simulink model "Robot_KinematicsSim_2019b1"  (R2020b)
settings: Solver=VariableStepAuto  StartTime=0.0  StopTime=1000  RelTol=1e-3  EnableMultiTasking=on
model workspace (MAT data in the model file):
  Ts = 0.01
  Xmax = 500
  Ymax = 500
values from neighbouring files (symbols this model uses):
  animation_update_interval = C*h_fixed    [setup.m]
  enable_CG_trace = 1    [setup.m]
  enable_rearAxle_trace = 0    [setup.m]
  plotAxisLimitMode = 0    [setup.m]
  plotAxisLimits = plotAxisLimits    [graphical_development.m]    (also in setup.m = [-3 5 -3 6]*3)
  save_anim_frames = 0    [setup.m]
  vehicle_length = 5    [setup.m]
  vehicle_width = 2    [setup.m]
undefined symbols (not defined in the file or in its folder): datetime, DiscIntNeverNeededParam
libraries: arduinolib x21, simulink x4, pid_lib x2
(part 1 of 2)
settings Model: SimulationMode=accelerator  SILPILModeSetting=veronly  PacingRate=89  ExtModeTrigDuration=2  Creator=pc world  LastModifiedBy=Omen
settings SolverCC: AutoInsertRateTranBlk=on
settings OptimizationCC: EnhancedBackFolding=on  PassReuseOutputArgsAs=Individual arguments  ZeroExternalMemoryAtStartup=off  ZeroInternalMemoryAtStartup=off  MaxStackSize=64  OptimizeBlockOrder=speed  DifferentSizesBufferReuse=on  OptimizationCustomize=off  EfficientTunableParamExpr=on
settings DebuggingCC: ParameterTunabilityLossMsg=error  SFUnexpectedBacktrackingDiag=warning  SFNoUnconditionalDefaultTransitionDiag=warning  UnderSpecifiedDimensionMsg=warning
settings HardwareCC: ProdBitPerInt=16  ProdBitPerPointer=16  ProdBitPerSizeT=16  ProdBitPerPtrDiffT=16  ProdLargestAtomicFloat=None  ProdWordSize=8  ProdHWDeviceType=Atmel->AVR
settings SFSimCC: MATLABDynamicMemAlloc=off
settings RTWCC: Description=Embedded Coder  SystemTargetFile=ert.tlc  HardwareBoard=Arduino Uno  TemplateMakefile=ert_default_tmf  GenerateReport=on  Toolchain=Arduino AVR  BuildConfiguration=Faster Runs  LaunchReport=on
settings CodeAppCC: ForceParamTrailComments=on  IgnoreCustomStorageClasses=off  OperatorAnnotations=on  SimulinkDataObjDesc=on  SFDataObjDesc=on  InsertBlockDesc=on
settings ERTTargetCC: SupportContinuousTime=on  SupportVariableSizeSignals=on  ExtMode=on  ExtModeStaticAllocSize=250  ExtModeMexArgs='127.0.0.1' 0 17725

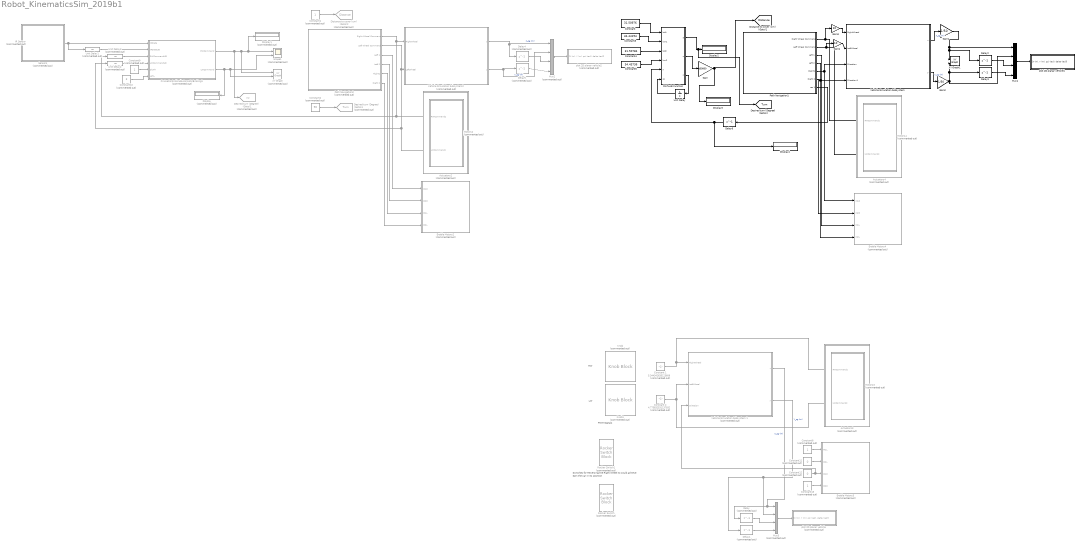
== system Robot_KinematicsSim_2019b1 ==
  note: PWM Signals
  note: RW
  note: LW
  note: Switches for Reversing the Right Wheel
      | to could achieve Spin the car in its position
  Actuators2 : Subsystem  Commented=on
  Actuators3 : Subsystem  Commented=on
  Actuators4 : Subsystem  Commented=on
  Constant : Constant  Value=31.50976
  Constant 1 : Constant  Commented=on  Value=5.344342635123609
  Constant 2 : Constant  Commented=on  Value=4.775832531137932
  Constant1 : Constant  Commented=on
  Constant10 : Constant  Commented=on  Value=3  OutDataTypeStr=double  SampleTime=Ts
  Constant11 : Constant  Commented=on  Value=0
  Constant12 : Constant  Commented=on  Value=0
  Constant13 : Constant  Commented=on
  Constant2 : Constant  Commented=on  Value=90
  Constant3 : Constant  Value=34.44194
  Constant4 : Constant  Value=31.50784
  Constant5 : Constant  Value=34.43736
  Constant8 : Constant  Commented=on
  Constant9 : Constant  Commented=on  OutDataTypeStr=double  SampleTime=Ts
  CruiseControlAndAutomaticBraking1 : Stateflow chart  Commented=on  TreatAsAtomicUnit=on
  Delay{,1,4..5} (4 alike) : Delay  Commented=on  DelayLength=1
  Delay2 : Delay  DelayLength=1
  Delay3 : Delay  DelayLength=1
  Delay6 : Delay  DelayLength=1
  Desired turn (Degree) (Goto)1 : Goto  Commented=on  GotoTag=rw  TagVisibility=global
  Desired turn (Degree) (Goto)3 : Goto  Commented=on  GotoTag=Turn  TagVisibility=global
  Display : Display  Commented=on
  Display1 : Display  Commented=on
  Display2 : Display
  Display3 : Display
  Display4 : Display
  Distance to cover (cm) (Goto)2 : Goto  Commented=on  GotoTag=Distance  TagVisibility=global
  Enable Motors2 : Subsystem  Commented=on
  Enable Motors3 : Subsystem  Commented=on
  Enable Motors4 : Subsystem  Commented=on
  Gain : Gain  Gain=100000
  Gain1 : Gain  Gain=1/50
  Gain2 : Gain  Gain=1/50
  Gain3 : Gain  Gain=10
  Gain4 : Gain  Gain=10
  IR Sensor : Subsystem  Commented=on
  Knob : KnobBlock  Commented=on  ScaleMax=10
  Knob1 : KnobBlock  Commented=on  ScaleMax=10
  MATLAB Function : MATLAB Function  TreatAsAtomicUnit=on
  Motors2 : Subsystem  Commented=on
  Motors3 : Subsystem  Commented=on
  Motors4 : Subsystem  Commented=on
  Mux1 : Mux
  Mux2 : Mux  Commented=on
  Mux3 : Mux  Commented=on
  Path Navigation1 : Subsystem
  Path Navigation2 : Subsystem  Commented=on
  Rocker Switch : RockerSwitchBlock  Commented=on
      settings: Values={{'Off', 'On'}, [0 1]}
  Rocker Switch1 : RockerSwitchBlock  Commented=on
      settings: Values={{'Off', 'On'}, [0 1]}
  Scope1 : Scope  Commented=on  NumInputPorts=2
  Sensors : Subsystem  Commented=on
  Unit Delay : UnitDelay  SampleTime=-1  HasFrameUpgradeWarning=on
  Unit Delay1 : UnitDelay  Commented=on  SampleTime=0.5  HasFrameUpgradeWarning=on
  Unit Delay2 : UnitDelay  Commented=on  SampleTime=0.5  HasFrameUpgradeWarning=on
  Unit Delay3 : UnitDelay  Commented=on  SampleTime=0.5  HasFrameUpgradeWarning=on
  "Vehicle Simulation Subsystem " : Subsystem
  Vehicle Simulation Subsystem 1 : Subsystem  Commented=on
  Vehicle Simulation Subsystem2 : Subsystem  Commented=on
  XY Graph : simulink/Sinks/XY Graph  Commented=on  xmin=-500  xmax=500  ymin=-500  ymax=500  st=0.05
  XY Graph1 : simulink/Sinks/XY Graph  xmin=-1000  xmax=1000  ymin=-1000  ymax=1000  st=0.05
  plot 2D planar vehicle : Subsystem  Commented=on  mask(6DoF Animation){axisMode=plotAxisLimitMode, ax=plotAxisLimits, Ts=animation_update_interval, enable_CG_trace=enable_CG_trace, enable_rearAxle_trace=enable_rearAxle_trace, save_anim_frames=save_anim_frames, anim_frame_name_str=char(datetime('now','Format','yyyy-MM-dd_HH_mm_ss')), L=vehicle_length, W=vehicle_width}
      mask prompts: axisMode "Axis Mode (0->auto, 1->fixed, BOTH use Axes Limits below)"; ax "Axes limits [xmin xmax ymin ymax] (m):"; Ts "Time interval between updates (s):"; enable_CG_trace "Enable vehicle CG trace? (0/1)"; enable_rearAxle_trace "Enable rear axle trace? (0/1)"; save_anim_frames "Save animaton frames? (0/1)"; anim_frame_name_str "Animation sequence name (if save frames==1)"; L "Vehicle length (m)"; W "Vehicle width (m)"
      mask help:
      | Create a 2D animated view of a steering vehicle model with tires.
      |
      | Marc Compere
      | CompereM@saic.com
      | created : 22 August 2002
      | modified: 28 Dec 2015
      mask init:
      | Config.axisMode=axisMode;
      | Config.ax=ax;
      | Config.Ts=Ts;
      | Config.enable_CG_trace=enable_CG_trace;
      | Config.enable_rearAxle_trace=enable_rearAxle_trace;
      | Config.save_anim_frames=save_anim_frames;
      | Config.anim_frame_name_str=anim_frame_name_str;
      | Config.L=L;
      | Config.W=W;
      mask Help:
      | <p>This block generates a 3 dimensional display of a simulation trajectory, with the craft orientation displayed during flight</p>
      | 
      | <p>There are two inputs to this block, Position and Euler.  These inputs contain more than one signal as described below.</p>
      | 
      | <p><H4>Block Vector Input - Position</H4>
      | <ul>
      | <li>X Position</li>
      | <li>Y Position</li>
      | <li>Z Position</li>
      | </ul>
      | </p>
      | 
      | <p><H4>Block Vector Input - Euler</H4>
      |     <ul>
      |     <li>Roll Attitude</li>
      |     <li>Pitch Attitude</li>
      |     <li>Yaw Attitude</li>
      |    </ul>
      |    </p>
  plot 2D planar vehicle1 : Subsystem  mask(6DoF Animation){axisMode=plotAxisLimitMode, ax=[-500 500 -500 500], Ts=animation_update_interval, enable_CG_trace=enable_CG_trace, enable_rearAxle_trace=enable_rearAxle_trace, save_anim_frames=save_anim_frames, anim_frame_name_str=char(datetime('now','Format','yyyy-MM-dd_HH_mm_ss')), L=vehicle_length, W=vehicle_width}
      mask prompts: axisMode "Axis Mode (0->auto, 1->fixed, BOTH use Axes Limits below)"; ax "Axes limits [xmin xmax ymin ymax] (m):"; Ts "Time interval between updates (s):"; enable_CG_trace "Enable vehicle CG trace? (0/1)"; enable_rearAxle_trace "Enable rear axle trace? (0/1)"; save_anim_frames "Save animaton frames? (0/1)"; anim_frame_name_str "Animation sequence name (if save frames==1)"; L "Vehicle length (m)"; W "Vehicle width (m)"
      mask help:
      | Create a 2D animated view of a steering vehicle model with tires.
      |
      | Marc Compere
      | CompereM@saic.com
      | created : 22 August 2002
      | modified: 28 Dec 2015
      mask init: same as Robot_KinematicsSim_2019b1/plot 2D planar vehicle
      mask Help:
      | <p>This block generates a 3 dimensional display of a simulation trajectory, with the craft orientation displayed during flight</p>
      | 
      | <p>There are two inputs to this block, Position and Euler.  These inputs contain more than one signal as described below.</p>
      | 
      | <p><H4>Block Vector Input - Position</H4>
      | <ul>
      | <li>X Position</li>
      | <li>Y Position</li>
      | <li>Z Position</li>
      | </ul>
      | </p>
      | 
      | <p><H4>Block Vector Input - Euler</H4>
      |     <ul>
      |     <li>Roll Attitude</li>
      |     <li>Pitch Attitude</li>
      |     <li>Yaw Attitude</li>
      |    </ul>
      |    </p>
  plot 2D planar vehicle2 : Subsystem  Commented=on  mask(6DoF Animation){axisMode=plotAxisLimitMode, ax=plotAxisLimits, Ts=animation_update_interval, enable_CG_trace=enable_CG_trace, enable_rearAxle_trace=enable_rearAxle_trace, save_anim_frames=save_anim_frames, anim_frame_name_str=char(datetime('now','Format','yyyy-MM-dd_HH_mm_ss')), L=vehicle_length, W=vehicle_width}
      mask prompts: axisMode "Axis Mode (0->auto, 1->fixed, BOTH use Axes Limits below)"; ax "Axes limits [xmin xmax ymin ymax] (m):"; Ts "Time interval between updates (s):"; enable_CG_trace "Enable vehicle CG trace? (0/1)"; enable_rearAxle_trace "Enable rear axle trace? (0/1)"; save_anim_frames "Save animaton frames? (0/1)"; anim_frame_name_str "Animation sequence name (if save frames==1)"; L "Vehicle length (m)"; W "Vehicle width (m)"
      mask help:
      | Create a 2D animated view of a steering vehicle model with tires.
      |
      | Marc Compere
      | CompereM@saic.com
      | created : 22 August 2002
      | modified: 28 Dec 2015
      mask init: same as Robot_KinematicsSim_2019b1/plot 2D planar vehicle
      mask Help:
      | <p>This block generates a 3 dimensional display of a simulation trajectory, with the craft orientation displayed during flight</p>
      | 
      | <p>There are two inputs to this block, Position and Euler.  These inputs contain more than one signal as described below.</p>
      | 
      | <p><H4>Block Vector Input - Position</H4>
      | <ul>
      | <li>X Position</li>
      | <li>Y Position</li>
      | <li>Z Position</li>
      | </ul>
      | </p>
      | 
      | <p><H4>Block Vector Input - Euler</H4>
      |     <ul>
      |     <li>Roll Attitude</li>
      |     <li>Pitch Attitude</li>
      |     <li>Yaw Attitude</li>
      |    </ul>
      |    </p>
  tag scope: Distance=global, Turn=global
  wires:
  Constant 1/1 -> Motors3/1(RWCommands), Vehicle Simulation Subsystem 1/1(RightWheel)
  Constant 2/1 -> Motors3/2(LWCommands), Vehicle Simulation Subsystem 1/2(LeftWheel)
  CruiseControlAndAutomaticBraking1/2(LWCommand) -> Scope1/2, XY Graph/2, Display/1
  CruiseControlAndAutomaticBraking1/1(RWCommand) -> Desired turn (Degree) (Goto)1/1, Scope1/1, Display1/1, XY Graph/1
  Unit Delay1/1 -> CruiseControlAndAutomaticBraking1/2(IRDataUD)
  Constant10/1 -> CruiseControlAndAutomaticBraking1/6(IRTh)
  IR Sensor/1(IRSensorMeasurement) -> Unit Delay1/1, CruiseControlAndAutomaticBraking1/1(IRData)
  Constant9/1 -> CruiseControlAndAutomaticBraking1/5(DisTh)
  Unit Delay3/1 -> CruiseControlAndAutomaticBraking1/3(RWCommandUD)
  Unit Delay2/1 -> CruiseControlAndAutomaticBraking1/4(LWCommandUD)
  Constant12/1 -> Enable Motors3/3(IN1R), Vehicle Simulation Subsystem 1/3(Direction)
  Constant8/1 -> Enable Motors3/1(IN1L)
  Constant13/1 -> Enable Motors3/4(IN2R)
  Constant11/1 -> Enable Motors3/2(IN2L)
  Mux3/1 -> plot 2D planar vehicle/1("[X (m), Y (m), psi (rad), delta (rad)]")
  Delay1/1 -> Mux3/4
  Delay/1 -> Mux3/3
  Vehicle Simulation Subsystem 1/1(x) -> Mux3/1, Delay/1  "X_cg (m)"
  Vehicle Simulation Subsystem 1/2(y) -> Mux3/2, Delay1/1  "Y_cg (m)"
  MATLAB Function/1(a) -> [Turn], Display2/1
  Path Navigation1/2(Left Wheel Command) -> Gain4/1, Motors4/2(LWCommands)
  Path Navigation1/1(Right Wheel Command) -> Gain3/1, Motors4/1(RWCommands)
  Delay2/1 -> Mux1/3
  Mux1/1 -> plot 2D planar vehicle1/1("[X (m), Y (m), psi (rad), delta (rad)]")
  Mux2/1 -> plot 2D planar vehicle2/1("[X (m), Y (m), psi (rad), delta (rad)]")
  Delay5/1 -> Mux2/4
  Delay4/1 -> Mux2/3
  Vehicle Simulation Subsystem2/1(x) -> Mux2/1, Delay4/1  "X_cg (m)"
  Vehicle Simulation Subsystem2/2(y) -> Mux2/2, Delay5/1  "Y_cg (m)"
  Path Navigation2/1(Right Wheel Command) -> Vehicle Simulation Subsystem2/1(RightWheel), Motors2/1(RWCommands), Unit Delay3/1
  Path Navigation2/2(Left Wheel Command) -> Vehicle Simulation Subsystem2/2(LeftWheel), Unit Delay2/1, Motors2/2(LWCommands)
  Constant1/1 -> Distance to cover (cm) (Goto)2/1
  Constant2/1 -> Desired turn (Degree) (Goto)3/1
  Path Navigation2/3(Left 1) -> Enable Motors2/1(IN1R)
  Path Navigation2/4(Left 2) -> Enable Motors2/2(IN2R)
  Path Navigation2/5(Right1) -> Enable Motors2/3(IN1L)
  Path Navigation2/6(Right 2) -> Enable Motors2/4(IN2L)
  Delay3/1 -> Mux1/4
  Path Navigation1/5(Right1) -> Enable Motors4/1(IN1R), "Vehicle Simulation Subsystem "/3(Direction)
  Path Navigation1/3(Left 1) -> Enable Motors4/3(IN1L)
  Path Navigation1/4(Left 2) -> Enable Motors4/4(IN2L), "Vehicle Simulation Subsystem "/4(Direction1)
  Path Navigation1/6(Right 2) -> Enable Motors4/2(IN2R)
  Constant4/1 -> MATLAB Function/3(lat2)
  Constant5/1 -> MATLAB Function/4(lon2)
  Unit Delay/1 -> MATLAB Function/6(ss)
  MATLAB Function/3(s) -> Unit Delay/1
  Constant/1 -> MATLAB Function/1(lat1)
  Constant3/1 -> MATLAB Function/2(lon1)
  Path Navigation1/7(res 1) -> Delay6/1
  Delay6/1 -> Display4/1, MATLAB Function/5(n)
  MATLAB Function/2(c) -> Gain/1
  Gain/1 -> [Distance], Display3/1
  "Vehicle Simulation Subsystem "/1(x) -> Gain1/1  "X_cg (m)"
  Gain1/1 -> Mux1/1, XY Graph1/1, Delay2/1
  "Vehicle Simulation Subsystem "/2(y) -> Gain2/1  "Y_cg (m)"
  Gain2/1 -> Delay3/1, XY Graph1/2, Mux1/2
  Gain3/1 -> "Vehicle Simulation Subsystem "/1(RightWheel)
  Gain4/1 -> "Vehicle Simulation Subsystem "/2(LeftWheel)

== system Robot_KinematicsSim_2019b1/Actuators2 ==

== system Robot_KinematicsSim_2019b1/Actuators3 ==

== system Robot_KinematicsSim_2019b1/Actuators4 ==

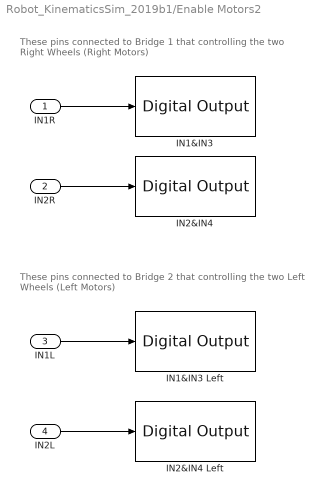
== system Robot_KinematicsSim_2019b1/Enable Motors2 ==
  note: These pins connected to Bridge 1 that
      | controlling the two Right Wheels (Right Motors)
  note: These pins connected to Bridge 2 that
      | controlling the two Left Wheels (Left Motors)
  IN1R : Inport
  IN2R : Inport  Port=2
  IN1L : Inport  Port=3
  IN2L : Inport  Port=4
  IN1&IN3 : arduinolib/Digital Output  pinNumber=12  Direction=output  blockPlatform=arduino
  IN1&IN3 Left : arduinolib/Digital Output  pinNumber=8  Direction=output  blockPlatform=arduino
  IN2&IN4 : arduinolib/Digital Output  pinNumber=4  Direction=output  blockPlatform=arduino
  IN2&IN4 Left : arduinolib/Digital Output  pinNumber=7  Direction=output  blockPlatform=arduino
  wires:
  IN2R/1 -> IN2&IN4/1
  IN1R/1 -> IN1&IN3/1
  IN1L/1 -> IN1&IN3 Left/1
  IN2L/1 -> IN2&IN4 Left/1

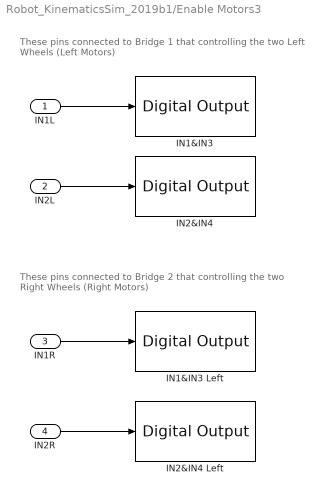
== system Robot_KinematicsSim_2019b1/Enable Motors3 ==
  note: These pins connected to Bridge 1 that
      | controlling the two Left Wheels (Left Motors)
  note: These pins connected to Bridge 2 that
      | controlling the two Right Wheels (Right Motors)
  IN1L : Inport
  IN2L : Inport  Port=2
  IN1R : Inport  Port=3
  IN2R : Inport  Port=4
  IN1&IN3 : arduinolib/Digital Output  pinNumber=12  Direction=output  blockPlatform=arduino
  IN1&IN3 Left : arduinolib/Digital Output  pinNumber=8  Direction=output  blockPlatform=arduino
  IN2&IN4 : arduinolib/Digital Output  pinNumber=4  Direction=output  blockPlatform=arduino
  IN2&IN4 Left : arduinolib/Digital Output  pinNumber=7  Direction=output  blockPlatform=arduino
  wires:
  IN2L/1 -> IN2&IN4/1
  IN1L/1 -> IN1&IN3/1
  IN1R/1 -> IN1&IN3 Left/1
  IN2R/1 -> IN2&IN4 Left/1

== system Robot_KinematicsSim_2019b1/Enable Motors4 ==
  note: These pins connected to Bridge 2 that
      | controlling the two Left Wheels (Left Motors)
  note: These pins connected to Bridge 1 that
      | controlling the two Right Wheels (Right Motors)
  IN1R : Inport
  IN2R : Inport  Port=2
  IN1L : Inport  Port=3
  IN2L : Inport  Port=4
  IN1&IN3 : arduinolib/Digital Output  pinNumber=12  Direction=output  blockPlatform=arduino
  IN1&IN3 Left : arduinolib/Digital Output  pinNumber=8  Direction=output  blockPlatform=arduino
  IN2&IN4 : arduinolib/Digital Output  pinNumber=4  Direction=output  blockPlatform=arduino
  IN2&IN4 Left : arduinolib/Digital Output  pinNumber=7  Direction=output  blockPlatform=arduino
  wires:
  IN2R/1 -> IN2&IN4 Left/1
  IN1R/1 -> IN1&IN3 Left/1
  IN1L/1 -> IN1&IN3/1
  IN2L/1 -> IN2&IN4/1

== system Robot_KinematicsSim_2019b1/IR Sensor ==
  "1-D Lookup Table " : Lookup_n-D  NumberOfTableDimensions=1  BreakpointsForDimension1=[440 470 500 550 700 850 1300 2250]  Table=[80 70 60 50 40 30 20 10]  ExtrapMethod=Clip  UseLastTableValue=on  InternalRulePriority=Speed  OutDataTypeStr=double  RndMeth=Simplest  InputSameDT=on
  "Analog Input " : arduinolib/Analog Input  pinNumber=4  ReadResultsOnly=off  ConversionTriggerSource=Software  ExternalTriggerType=uint32(0)  OutputDataType=uint16  EnableConversionCompleteNotify=off  EnableOuputStatus=off  SampleTime=Ts  blockPlatform=arduino
  Conversion to mV : Gain  Gain=3300/1023  OutDataTypeStr=int16
  "Discrete Transfer Fcn " : DiscreteTransferFcn  Numerator=0.5  Denominator=[1 -0.5]  OutDataTypeStr=int16
  Mux : Mux  Inputs=2
  Scope1 : Scope
  Scope2 : Scope
  IRSensorMeasurement : Outport
  wires:
  "Analog Input "/1 -> Conversion to mV/1
  Mux/1 -> Scope1/1
  Conversion to mV/1 -> "Discrete Transfer Fcn "/1, Mux/2  "raw Signal"
  "1-D Lookup Table "/1 -> Scope2/1, IRSensorMeasurement/1
  "Discrete Transfer Fcn "/1 -> Mux/1, "1-D Lookup Table "/1  "filtered Signal"

== system Robot_KinematicsSim_2019b1/Motors2 ==
  note: 10 is the maximum input from our model system
      | after scaling by 25.5 ,it will be equal 255
  RWCommands : Inport
  LWCommands : Inport  Port=2
  PWM to Enable the Left Bridge : arduinolib/PWM  pinNumber=6  frequencyType=Default  desiredFrequency=490.2  achievableFrequency=490.2
  PWM to Enable the Right Bridge : arduinolib/PWM  pinNumber=5  frequencyType=Default  desiredFrequency=490.2  achievableFrequency=490.2
  Scale1 : Gain  Gain=25.5
  Scale2 : Gain  Gain=25.5
  wires:
  LWCommands/1 -> Scale2/1
  RWCommands/1 -> Scale1/1
  Scale2/1 -> PWM to Enable the Left Bridge/1
  Scale1/1 -> PWM to Enable the Right Bridge/1

== system Robot_KinematicsSim_2019b1/Motors3 ==
  note: 10 is the maximum input from our model system
      | after scaling by 25.5 ,it will be equal 255
  RWCommands : Inport
  LWCommands : Inport  Port=2
  PWM to Enable the Left Bridge : arduinolib/PWM  pinNumber=6  frequencyType=Default  desiredFrequency=490.2  achievableFrequency=490.2
  PWM to Enable the Right Bridge : arduinolib/PWM  pinNumber=5  frequencyType=Default  desiredFrequency=490.2  achievableFrequency=490.2
  Scale1 : Gain  Gain=25.5
  Scale2 : Gain  Gain=25.5
  wires:
  LWCommands/1 -> Scale2/1
  RWCommands/1 -> Scale1/1
  Scale2/1 -> PWM to Enable the Left Bridge/1
  Scale1/1 -> PWM to Enable the Right Bridge/1

== system Robot_KinematicsSim_2019b1/Motors4 ==
  note: 10 is the maximum input from our model system
      | after scaling by 25.5 ,it will be equal 255
  RWCommands : Inport
  LWCommands : Inport  Port=2
  PWM to Enable the Left Bridge : arduinolib/PWM  pinNumber=6  frequencyType=Default  desiredFrequency=490.2  achievableFrequency=490.2
  PWM to Enable the Right Bridge : arduinolib/PWM  pinNumber=5  frequencyType=Default  desiredFrequency=490.2  achievableFrequency=490.2
  Scale1 : Gain  Gain=25.5
  Scale2 : Gain  Gain=25.5
  wires:
  Scale1/1 -> PWM to Enable the Right Bridge/1
  Scale2/1 -> PWM to Enable the Left Bridge/1
  RWCommands/1 -> Scale1/1
  LWCommands/1 -> Scale2/1

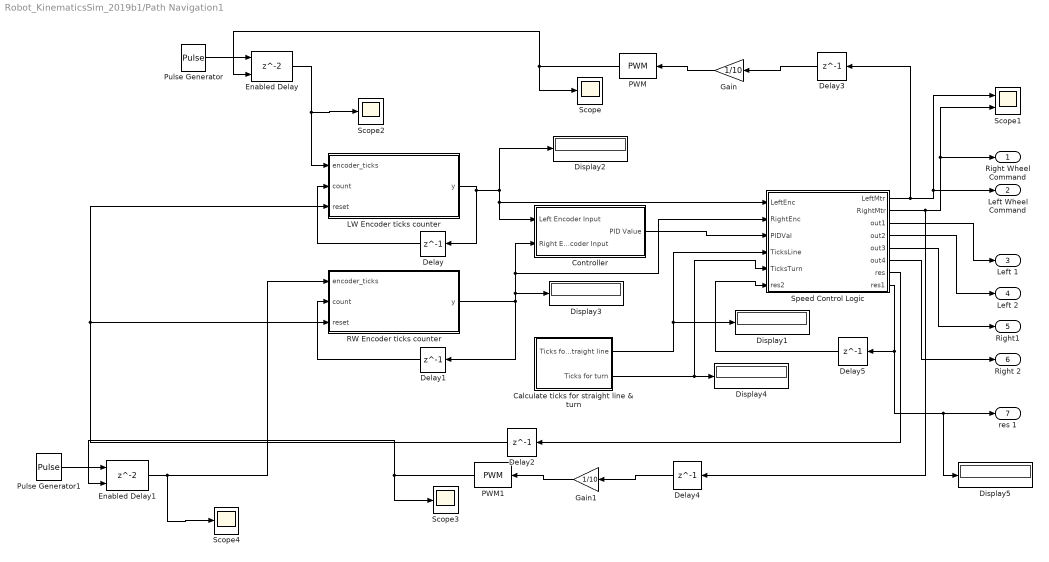
== system Robot_KinematicsSim_2019b1/Path Navigation1 ==
  Calculate ticks for straight line & turn : Subsystem
  Controller : Subsystem
  Delay{,1..2,5} (4 alike) : Delay  DelayLength=1  InitialCondition=0
  Delay3 : Delay  DelayLength=1
  Delay4 : Delay  DelayLength=1
  Display{1..5} (5 alike) : Display
  Enabled Delay : Delay  ShowEnablePort=on
      settings: InputPortMap=u0,e6
  Enabled Delay1 : Delay  ShowEnablePort=on
      settings: InputPortMap=u0,e6
  Gain : Gain  Gain=1/10
  Gain1 : Gain  Gain=1/10
  LW Encoder ticks counter : MATLAB Function  TreatAsAtomicUnit=on
  PWM : simulink/Discontinuities/PWM  DisableCoverage=on  Period=1/100  DisallowZeroDutyCycle=off  RunAtFixedTimeIntervals=on  SampleTime=0.01
  PWM1 : simulink/Discontinuities/PWM  DisableCoverage=on  Period=1/100  DisallowZeroDutyCycle=off  RunAtFixedTimeIntervals=on  SampleTime=0.01
  Pulse Generator : DiscretePulseGenerator  PulseType=Time based  Period=1/1000  PulseWidth=10  SampleTime=6
  Pulse Generator1 : DiscretePulseGenerator  PulseType=Time based  Period=1/1000  PulseWidth=10  SampleTime=6
  RW Encoder ticks counter : MATLAB Function  TreatAsAtomicUnit=on
  Scope{,2..4} (4 alike) : Scope
  Scope1 : Scope  NumInputPorts=2
  Speed Control Logic : MATLAB Function  TreatAsAtomicUnit=on
      settings: CopyFcn=set_param(gcb, 'LinkStatus', 'none') ;
  Right Wheel Command : Outport
  Left Wheel Command : Outport  Port=2
  Left 1 : Outport  Port=3
  Left 2 : Outport  Port=4
  Right1 : Outport  Port=5
  Right 2 : Outport  Port=6
  res 1 : Outport  Port=7
  wires:
  Delay5/1 -> Speed Control Logic/6(res2)
  Speed Control Logic/6(out4) -> Right 2/1
  Speed Control Logic/5(out3) -> Right1/1
  Speed Control Logic/4(out2) -> Left 2/1
  Speed Control Logic/3(out1) -> Left 1/1
  Delay2/1 -> LW Encoder ticks counter/3(reset), RW Encoder ticks counter/3(reset)
  Speed Control Logic/7(res) -> Delay2/1
  Enabled Delay1/1 -> RW Encoder ticks counter/1(encoder_ticks), Scope4/1
  RW Encoder ticks counter/1(y) -> Display3/1, Speed Control Logic/2(RightEnc), Controller/2(Right Encoder Input), Delay1/1
  Delay1/1 -> RW Encoder ticks counter/2(count)
  Delay/1 -> LW Encoder ticks counter/2(count)
  LW Encoder ticks counter/1(y) -> Speed Control Logic/1(LeftEnc), Controller/1(Left Encoder Input), Display2/1, Delay/1
  Speed Control Logic/2(RightMtr) -> Delay4/1, Scope1/2, Right Wheel Command/1
  Calculate ticks for straight line & turn/1("Ticks for straight line ") -> Speed Control Logic/4(TicksLine), Display1/1
  Controller/1(PID Value) -> Speed Control Logic/3(PIDVal)
  Speed Control Logic/1(LeftMtr) -> Delay3/1, Left Wheel Command/1, Scope1/1
  Calculate ticks for straight line & turn/2(Ticks for turn) -> Display4/1, Speed Control Logic/5(TicksTurn)
  Speed Control Logic/8(res1) -> Delay5/1, Display5/1, res 1/1
  Enabled Delay/1 -> Scope2/1, LW Encoder ticks counter/1(encoder_ticks)
  Pulse Generator/1 -> Enabled Delay/1
  Gain/1 -> PWM/1
  PWM/1 -> Scope/1, Enabled Delay/2
  Delay3/1 -> Gain/1
  Gain1/1 -> PWM1/1
  Delay4/1 -> Gain1/1
  Pulse Generator1/1 -> Enabled Delay1/1
  PWM1/1 -> Scope3/1, Enabled Delay1/2

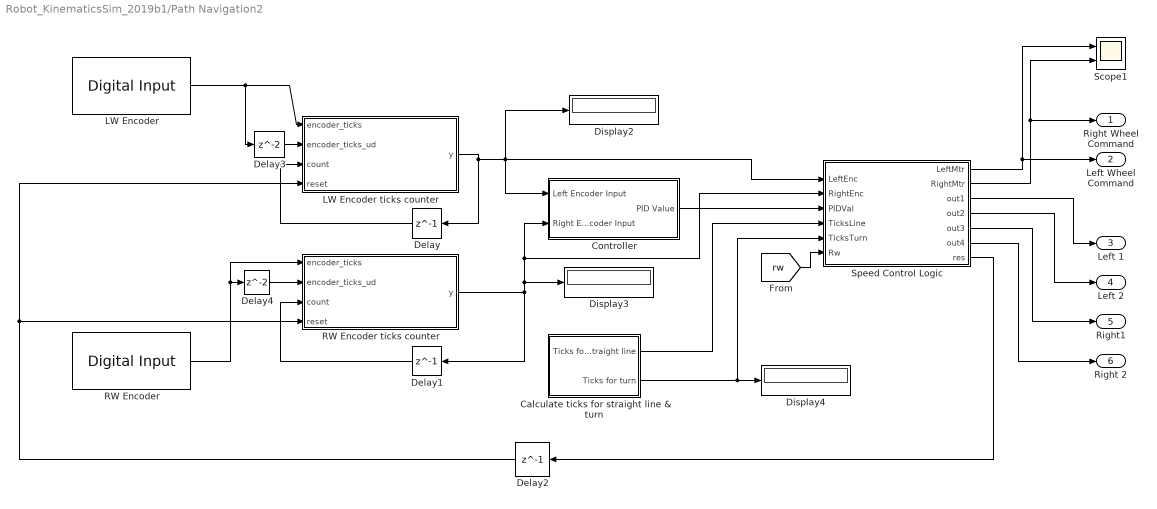
== system Robot_KinematicsSim_2019b1/Path Navigation2 ==
  Calculate ticks for straight line & turn : Subsystem
  Controller : Subsystem
  Delay : Delay  DelayLength=1  InitialCondition=0
  Delay1 : Delay  DelayLength=1  InitialCondition=0
  Delay2 : Delay  DelayLength=1  InitialCondition=0
  Delay3 : Delay  InitialCondition=0
  Delay4 : Delay  InitialCondition=0
  Display2 : Display
  Display3 : Display
  Display4 : Display
  LW Encoder : arduinolib/Digital Input  pinNumber=2  mode=Default  Direction=input  SampleTime=0.1  blockPlatform=arduino
  LW Encoder ticks counter : MATLAB Function  TreatAsAtomicUnit=on
  RW Encoder : arduinolib/Digital Input  pinNumber=3  mode=Default  Direction=input  SampleTime=0.1  blockPlatform=arduino
  RW Encoder ticks counter : MATLAB Function  TreatAsAtomicUnit=on
  Scope1 : Scope  NumInputPorts=2
  Speed Control Logic : MATLAB Function  TreatAsAtomicUnit=on
      settings: CopyFcn=set_param(gcb, 'LinkStatus', 'none') ;
  Right Wheel Command : Outport
  Left Wheel Command : Outport  Port=2
  Left 1 : Outport  Port=3
  Left 2 : Outport  Port=4
  Right1 : Outport  Port=5
  Right 2 : Outport  Port=6
  wires:
  Calculate ticks for straight line & turn/2(Ticks for turn) -> Speed Control Logic/5(TicksTurn), Display4/1
  Speed Control Logic/1(LeftMtr) -> Scope1/1, Left Wheel Command/1
  Controller/1(PID Value) -> Speed Control Logic/3(PIDVal)
  Calculate ticks for straight line & turn/1("Ticks for straight line ") -> Speed Control Logic/4(TicksLine)
  Speed Control Logic/2(RightMtr) -> Right Wheel Command/1, Scope1/2
  LW Encoder ticks counter/1(y) -> Delay/1, Controller/1(Left Encoder Input), Speed Control Logic/1(LeftEnc), Display2/1
  LW Encoder/1 -> Delay3/1, LW Encoder ticks counter/1(encoder_ticks)
  Delay/1 -> LW Encoder ticks counter/3(count)
  Delay1/1 -> RW Encoder ticks counter/3(count)
  RW Encoder ticks counter/1(y) -> Delay1/1, Controller/2(Right Encoder Input), Speed Control Logic/2(RightEnc), Display3/1
  RW Encoder/1 -> Delay4/1, RW Encoder ticks counter/1(encoder_ticks)
  Speed Control Logic/7(res) -> Delay2/1
  Delay2/1 -> RW Encoder ticks counter/4(reset), LW Encoder ticks counter/4(reset)
  Speed Control Logic/3(out1) -> Left 1/1
  Speed Control Logic/4(out2) -> Left 2/1
  Speed Control Logic/5(out3) -> Right1/1
  Speed Control Logic/6(out4) -> Right 2/1
  Delay3/1 -> LW Encoder ticks counter/2(encoder_ticks_ud)
  Delay4/1 -> RW Encoder ticks counter/2(encoder_ticks_ud)
  [rw] -> Speed Control Logic/6(Rw)

== system Robot_KinematicsSim_2019b1/Sensors ==

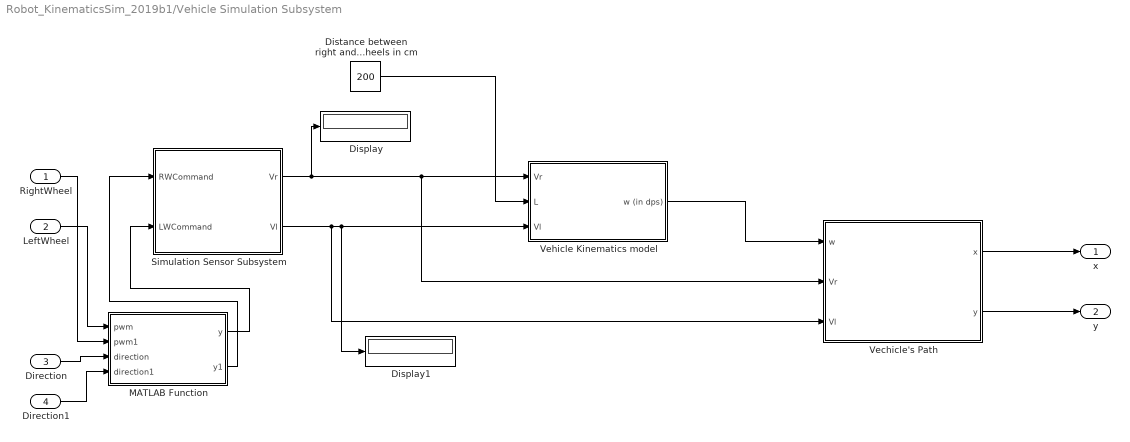
== system Robot_KinematicsSim_2019b1/Vehicle Simulation Subsystem  ==
  RightWheel : Inport
  LeftWheel : Inport  Port=2
  Direction : Inport  Port=3
  Direction1 : Inport  Port=4
  Display : Display
  Display1 : Display
  "Distance between right and left wheels in cm " : Constant  Value=200
  MATLAB Function : MATLAB Function  TreatAsAtomicUnit=on
  Simulation Sensor Subsystem : Subsystem
  "Vechicle's Path " : Subsystem
  "Vehicle Kinematics model " : Subsystem
  x : Outport
  y : Outport  Port=2
  wires:
  "Distance between right and left wheels in cm "/1 -> "Vehicle Kinematics model "/2(L)
  Simulation Sensor Subsystem/2(Vl) -> "Vehicle Kinematics model "/3("Vl "), Display1/1, "Vechicle's Path "/3(Vl)
  Simulation Sensor Subsystem/1(Vr) -> Display/1, "Vehicle Kinematics model "/1(Vr), "Vechicle's Path "/2(Vr)
  "Vechicle's Path "/2(y) -> y/1
  "Vechicle's Path "/1(x) -> x/1
  LeftWheel/1 -> MATLAB Function/1(pwm)
  MATLAB Function/1(y) -> Simulation Sensor Subsystem/2(LWCommand)
  Direction/1 -> MATLAB Function/3(direction)
  RightWheel/1 -> MATLAB Function/2(pwm1)
  MATLAB Function/2(y1) -> Simulation Sensor Subsystem/1(RWCommand)
  Direction1/1 -> MATLAB Function/4(direction1)
  "Vehicle Kinematics model "/1("w (in dps) ") -> "Vechicle's Path "/1(w)

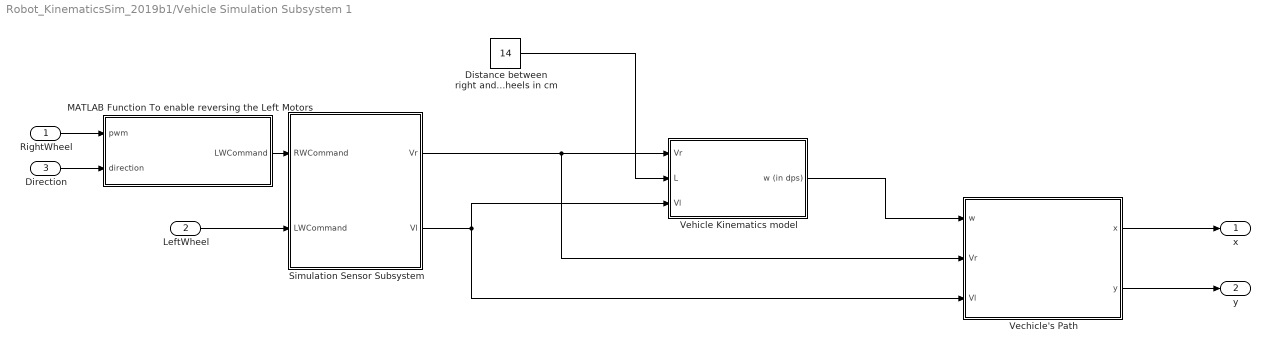
== system Robot_KinematicsSim_2019b1/Vehicle Simulation Subsystem 1 ==
  RightWheel : Inport
  LeftWheel : Inport  Port=2
  Direction : Inport  Port=3
  "Distance between right and left wheels in cm " : Constant  Value=14
  "MATLAB Function To enable reversing the Left Motors " : MATLAB Function  TreatAsAtomicUnit=on
  Simulation Sensor Subsystem : Subsystem
  "Vechicle's Path " : Subsystem
  "Vehicle Kinematics model " : Subsystem
  x : Outport
  y : Outport  Port=2
  wires:
  "Distance between right and left wheels in cm "/1 -> "Vehicle Kinematics model "/2(L)
  Simulation Sensor Subsystem/2(Vl) -> "Vechicle's Path "/3(Vl), "Vehicle Kinematics model "/3("Vl ")
  Simulation Sensor Subsystem/1(Vr) -> "Vechicle's Path "/2(Vr), "Vehicle Kinematics model "/1(Vr)
  "Vehicle Kinematics model "/1("w (in dps) ") -> "Vechicle's Path "/1(w)
  "Vechicle's Path "/2(y) -> y/1
  "Vechicle's Path "/1(x) -> x/1
  Direction/1 -> "MATLAB Function To enable reversing the Left Motors "/2(direction)
  LeftWheel/1 -> Simulation Sensor Subsystem/2(LWCommand)
  "MATLAB Function To enable reversing the Left Motors "/1(LWCommand) -> Simulation Sensor Subsystem/1(RWCommand)
  RightWheel/1 -> "MATLAB Function To enable reversing the Left Motors "/1(pwm)

== system Robot_KinematicsSim_2019b1/Vehicle Simulation Subsystem2 ==
  RightWheel : Inport
  LeftWheel : Inport  Port=2
  "Distance between right and left wheels in cm " : Constant  Value=14
  Simulation Sensor Subsystem : Subsystem
  "Vechicle's Path " : Subsystem
  "Vehicle Kinematics model " : Subsystem
  x : Outport
  y : Outport  Port=2
  wires:
  "Vehicle Kinematics model "/1("w (in dps) ") -> "Vechicle's Path "/1(w)
  RightWheel/1 -> Simulation Sensor Subsystem/1(RWCommand)
  Simulation Sensor Subsystem/1(Vr) -> "Vechicle's Path "/2(Vr), "Vehicle Kinematics model "/1(Vr)
  "Vechicle's Path "/1(x) -> x/1
  Simulation Sensor Subsystem/2(Vl) -> "Vechicle's Path "/3(Vl), "Vehicle Kinematics model "/3("Vl ")
  LeftWheel/1 -> Simulation Sensor Subsystem/2(LWCommand)
  "Distance between right and left wheels in cm "/1 -> "Vehicle Kinematics model "/2(L)
  "Vechicle's Path "/2(y) -> y/1

== system Robot_KinematicsSim_2019b1/plot 2D planar vehicle ==
  "[X (m), Y (m), psi (rad), delta (rad)]" : Inport
  Animation S-Function : S-Function  FunctionName=sanim_XY_vehicle_viz  Parameters=Config  SFunctionDeploymentMode=off  EnableBusSupport=off
  Rate Transition : RateTransition  Integrity=off
  wires:
  "[X (m), Y (m), psi (rad), delta (rad)]"/1 -> Rate Transition/1
  Rate Transition/1 -> Animation S-Function/1

== system Robot_KinematicsSim_2019b1/plot 2D planar vehicle1 ==
  "[X (m), Y (m), psi (rad), delta (rad)]" : Inport
  Animation S-Function : S-Function  FunctionName=sanim_XY_vehicle_viz  Parameters=Config  SFunctionDeploymentMode=off  EnableBusSupport=off
  Rate Transition : RateTransition  Integrity=off
  wires:
  Rate Transition/1 -> Animation S-Function/1
  "[X (m), Y (m), psi (rad), delta (rad)]"/1 -> Rate Transition/1

== system Robot_KinematicsSim_2019b1/plot 2D planar vehicle2 ==
  "[X (m), Y (m), psi (rad), delta (rad)]" : Inport
  Animation S-Function : S-Function  FunctionName=sanim_XY_vehicle_viz  Parameters=Config  SFunctionDeploymentMode=off  EnableBusSupport=off
  Rate Transition : RateTransition  Integrity=off
  wires:
  "[X (m), Y (m), psi (rad), delta (rad)]"/1 -> Rate Transition/1
  Rate Transition/1 -> Animation S-Function/1

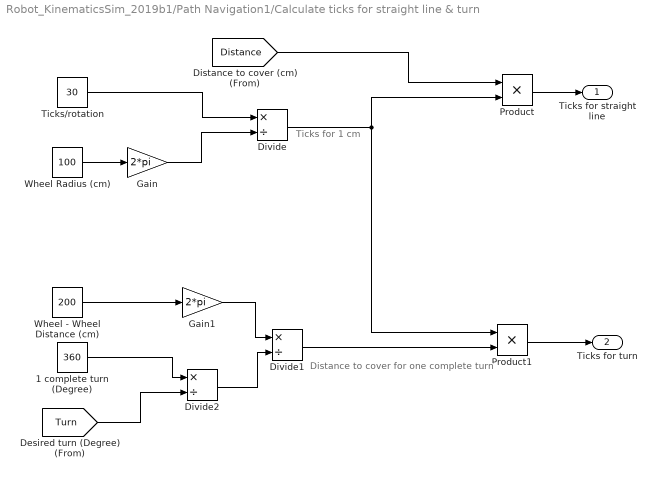
== system Robot_KinematicsSim_2019b1/Path Navigation1/Calculate ticks for straight line & turn ==
  note: Ticks for 1 cm
  note: Distance to cover for one complete turn
  " 1 complete turn (Degree)" : Constant  Value=360
  Divide : Product  Inputs=*/
  Divide1 : Product  Inputs=*/
  Divide2 : Product  Inputs=*/
  Gain : Gain  Gain=2*pi
  Gain1 : Gain  Gain=2*pi
  Product : Product
  Product1 : Product
  Ticks/rotation : Constant  Value=30
  Wheel - Wheel Distance (cm) : Constant  Value=200
  Wheel Radius (cm) : Constant  Value=100
  "Ticks for straight line " : Outport  VectorParamsAs1DForOutWhenUnconnected=off
  Ticks for turn : Outport  Port=2  VectorParamsAs1DForOutWhenUnconnected=off
  wires:
  Divide1/1 -> Product1/2
  Divide2/1 -> Divide1/2
  Gain1/1 -> Divide1/1
  [Turn] -> Divide2/2
  " 1 complete turn (Degree)"/1 -> Divide2/1
  Product1/1 -> Ticks for turn/1
  Wheel - Wheel Distance (cm)/1 -> Gain1/1
  Divide/1 -> Product/2, Product1/1
  [Distance] -> Product/1
  Product/1 -> "Ticks for straight line "/1
  Wheel Radius (cm)/1 -> Gain/1
  Gain/1 -> Divide/2
  Ticks/rotation/1 -> Divide/1

== system Robot_KinematicsSim_2019b1/Path Navigation1/Controller ==
  Left Encoder Input : Inport
  Right Encoder Input : Inport  Port=2
  "Abs " : Abs
  "Abs1 " : Abs
  "Add " : Sum  Inputs=+-
  Discrete PID Controller : pid_lib/PID Controller  Controller=PID  Form=Parallel  TimeDomain=Discrete-time  UseExternalTs=off  SampleTime=-1  IntegratorMethod=Forward Euler  FilterMethod=Forward Euler  ControllerParametersSource=internal  P=0.05  I=0.005  D=0.01  UseFilter=off  N=100  TunerSelectOption=Transfer Function Based (PID Tuner App)  InitialConditionSource=internal  InitialConditionForIntegrator=0  InitialConditionForFilter=0  DifferentiatorICPrevScaledInput=0  ExternalReset=none  TrackingMode=off  Kt=1  LimitOutput=off  SatLimitsSource=internal  UpperSaturationLimit=inf  LowerSaturationLimit=-inf  LinearizeAsGain=off  AntiWindupMode=none  Kb=1  POutMin=[]  POutMax=[]  IOutMin=[]  IOutMax=[]  DOutMin=[]  DOutMax=[]  NOutMin=[]  NOutMax=[]  SumOutMin=[]  SumOutMax=[]  SaturationOutMin=[]  SaturationOutMax=[]  PParamMin=[]  PParamMax=[]  IParamMin=[]  IParamMax=[]  DParamMin=[]  DParamMax=[]  NParamMin=[]  NParamMax=[]  KbParamMin=[]  KbParamMax=[]  KtParamMin=[]  KtParamMax=[]  KbOutMin=[]  KbOutMax=[]  KtOutMin=[]  KtOutMax=[]  IntegratorOutMin=[]  IntegratorOutMax=[]  FilterOutMin=[]  FilterOutMax=[]  SumI1OutMin=[]  SumI1OutMax=[]  SumI2OutMin=[]  SumI2OutMax=[]  SumI3OutMin=[]  SumI3OutMax=[]  SumI4OutMin=[]  SumI4OutMax=[]  SumDOutMin=[]  SumDOutMax=[]  DifferentiatorOutMin=[]  DifferentiatorOutMax=[]  FilterDiffOutCoefMin=[]  FilterDiffOutCoefMax=[]  ReciprocalOutMin=[]  ReciprocalOutMax=[]  SumDenOutMin=[]  SumDenOutMax=[]  SumNumOutMin=[]  SumNumOutMax=[]  DivideOutMin=[]  DivideOutMax=[]  UdiffTsProdOutMin=[]  UdiffTsProdOutMax=[]  NTsProdOutMin=[]  NTsProdOutMax=[]  UintegralTsProdOutMin=[]  UintegralTsProdOutMax=[]  UngainTsProdOutMin=[]  UngainTsProdOutMax=[]  IntegratorContinuousStateAttributes=''  IntegratorStateMustResolveToSignalObject=off  IntegratorRTWStateStorageClass=Auto  FilterContinuousStateAttributes=''  FilterStateMustResolveToSignalObject=off  FilterRTWStateStorageClass=Auto  ParallelPVariant=InternalParameters  IdealPVariant=Disabled  IVariant=InternalParameters  DVariant=InternalParameters  IntegratorVariant=Discrete  SatVariant=Disabled  AWVariant=Passthrough  PCopyVariant=Disabled  TRVariant=Disabled  FdbkBlocksVariant=Forward  IdealPFdbkVariant=Disabled  SatFdbkVariant=Disabled  DerivativeFilterVariant=Differentiator  NVariant=Passthrough  NCopyVariant=Disabled_SignalSpec  FilterICVariant=InternalICsDifferentiator  IntegratorICVariant=InternalICs  ExternalResetVariant=Disabled  TRSumVariant=Passthrough  SumFdbkVariant=Disabled  SumVariant=Sum_PID  TsampFilterVariant=InternalTs  TsampNgainVariant=Passthrough  TsampIntegralVariant=Passthrough  ExternalSaturationOutDataTypeStr=Inherit: Same as second input
  PID Value : Outport  VectorParamsAs1DForOutWhenUnconnected=off
  wires:
  Left Encoder Input/1 -> "Abs "/1
  Right Encoder Input/1 -> "Abs1 "/1
  Discrete PID Controller/1 -> PID Value/1
  "Abs "/1 -> "Add "/1
  "Abs1 "/1 -> "Add "/2
  "Add "/1 -> Discrete PID Controller/1

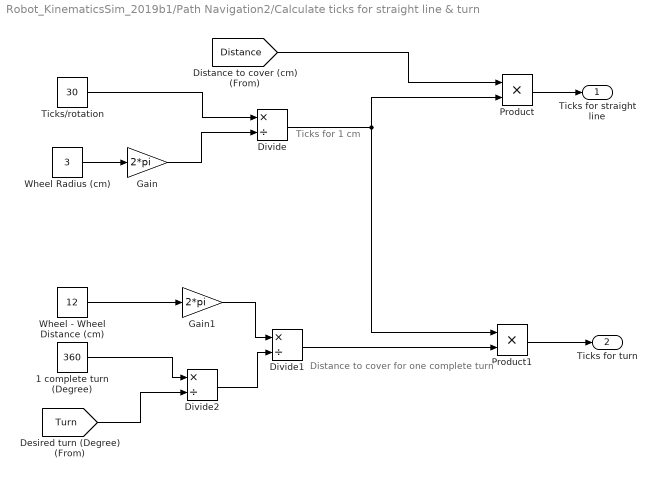
== system Robot_KinematicsSim_2019b1/Path Navigation2/Calculate ticks for straight line & turn ==
  note: Distance to cover for one complete turn
  note: Ticks for 1 cm
  " 1 complete turn (Degree)" : Constant  Value=360
  Divide : Product  Inputs=*/
  Divide1 : Product  Inputs=*/
  Divide2 : Product  Inputs=*/
  Gain : Gain  Gain=2*pi
  Gain1 : Gain  Gain=2*pi
  Product : Product
  Product1 : Product
  Ticks/rotation : Constant  Value=30
  Wheel - Wheel Distance (cm) : Constant  Value=12
  Wheel Radius (cm) : Constant  Value=3
  "Ticks for straight line " : Outport  VectorParamsAs1DForOutWhenUnconnected=off
  Ticks for turn : Outport  Port=2  VectorParamsAs1DForOutWhenUnconnected=off
  wires:
  Ticks/rotation/1 -> Divide/1
  Gain/1 -> Divide/2
  Wheel Radius (cm)/1 -> Gain/1
  Product/1 -> "Ticks for straight line "/1
  [Distance] -> Product/1
  Divide/1 -> Product1/1, Product/2
  Wheel - Wheel Distance (cm)/1 -> Gain1/1
  Product1/1 -> Ticks for turn/1
  " 1 complete turn (Degree)"/1 -> Divide2/1
  [Turn] -> Divide2/2
  Gain1/1 -> Divide1/1
  Divide2/1 -> Divide1/2
  Divide1/1 -> Product1/2

== system Robot_KinematicsSim_2019b1/Path Navigation2/Controller ==
  Left Encoder Input : Inport
  Right Encoder Input : Inport  Port=2
  "Abs " : Abs
  "Abs1 " : Abs
  "Add " : Sum  Inputs=+-
  Discrete PID Controller : pid_lib/PID Controller  Controller=PID  Form=Parallel  TimeDomain=Discrete-time  UseExternalTs=off  SampleTime=-1  IntegratorMethod=Forward Euler  FilterMethod=Forward Euler  ControllerParametersSource=internal  P=0.05  I=0.005  D=0.01  UseFilter=off  N=100  TunerSelectOption=Transfer Function Based (PID Tuner App)  InitialConditionSource=internal  InitialConditionForIntegrator=0  InitialConditionForFilter=0  DifferentiatorICPrevScaledInput=0  ExternalReset=none  TrackingMode=off  Kt=1  LimitOutput=off  SatLimitsSource=internal  UpperSaturationLimit=inf  LowerSaturationLimit=-inf  LinearizeAsGain=off  AntiWindupMode=none  Kb=1  POutMin=[]  POutMax=[]  IOutMin=[]  IOutMax=[]  DOutMin=[]  DOutMax=[]  NOutMin=[]  NOutMax=[]  SumOutMin=[]  SumOutMax=[]  SaturationOutMin=[]  SaturationOutMax=[]  PParamMin=[]  PParamMax=[]  IParamMin=[]  IParamMax=[]  DParamMin=[]  DParamMax=[]  NParamMin=[]  NParamMax=[]  KbParamMin=[]  KbParamMax=[]  KtParamMin=[]  KtParamMax=[]  KbOutMin=[]  KbOutMax=[]  KtOutMin=[]  KtOutMax=[]  IntegratorOutMin=[]  IntegratorOutMax=[]  FilterOutMin=[]  FilterOutMax=[]  SumI1OutMin=[]  SumI1OutMax=[]  SumI2OutMin=[]  SumI2OutMax=[]  SumI3OutMin=[]  SumI3OutMax=[]  SumI4OutMin=[]  SumI4OutMax=[]  SumDOutMin=[]  SumDOutMax=[]  DifferentiatorOutMin=[]  DifferentiatorOutMax=[]  FilterDiffOutCoefMin=[]  FilterDiffOutCoefMax=[]  ReciprocalOutMin=[]  ReciprocalOutMax=[]  SumDenOutMin=[]  SumDenOutMax=[]  SumNumOutMin=[]  SumNumOutMax=[]  DivideOutMin=[]  DivideOutMax=[]  UdiffTsProdOutMin=[]  UdiffTsProdOutMax=[]  NTsProdOutMin=[]  NTsProdOutMax=[]  UintegralTsProdOutMin=[]  UintegralTsProdOutMax=[]  UngainTsProdOutMin=[]  UngainTsProdOutMax=[]  IntegratorContinuousStateAttributes=''  IntegratorStateMustResolveToSignalObject=off  IntegratorRTWStateStorageClass=Auto  FilterContinuousStateAttributes=''  FilterStateMustResolveToSignalObject=off  FilterRTWStateStorageClass=Auto  ParallelPVariant=InternalParameters  IdealPVariant=Disabled  IVariant=InternalParameters  DVariant=InternalParameters  IntegratorVariant=Discrete  SatVariant=Disabled  AWVariant=Passthrough  PCopyVariant=Disabled  TRVariant=Disabled  FdbkBlocksVariant=Forward  IdealPFdbkVariant=Disabled  SatFdbkVariant=Disabled  DerivativeFilterVariant=Differentiator  NVariant=Passthrough  NCopyVariant=Disabled_SignalSpec  FilterICVariant=InternalICsDifferentiator  IntegratorICVariant=InternalICs  ExternalResetVariant=Disabled  TRSumVariant=Passthrough  SumFdbkVariant=Disabled  SumVariant=Sum_PID  TsampFilterVariant=InternalTs  TsampNgainVariant=Passthrough  TsampIntegralVariant=Passthrough  ExternalSaturationOutDataTypeStr=Inherit: Same as second input
  PID Value : Outport  VectorParamsAs1DForOutWhenUnconnected=off
  wires:
  "Add "/1 -> Discrete PID Controller/1
  "Abs1 "/1 -> "Add "/2
  "Abs "/1 -> "Add "/1
  Discrete PID Controller/1 -> PID Value/1
  Right Encoder Input/1 -> "Abs1 "/1
  Left Encoder Input/1 -> "Abs "/1

== system Robot_KinematicsSim_2019b1/Vehicle Simulation Subsystem /Simulation Sensor Subsystem ==
  RWCommand : Inport
  LWCommand : Inport  Port=2
  Conversion to Radians per s : Gain  Gain=2*pi/60
  Conversion to Radians per s1 : Gain  Gain=2*pi/60
  "Wheel Radius in cm " : Gain  Gain=100
  "Wheel Radius in cm1 " : Gain  Gain=100
  Vr : Outport
  Vl : Outport  Port=2
  wires:
  LWCommand/1 -> Conversion to Radians per s1/1
  RWCommand/1 -> Conversion to Radians per s/1
  "Wheel Radius in cm "/1 -> Vr/1
  "Wheel Radius in cm1 "/1 -> Vl/1
  Conversion to Radians per s1/1 -> "Wheel Radius in cm1 "/1
  Conversion to Radians per s/1 -> "Wheel Radius in cm "/1

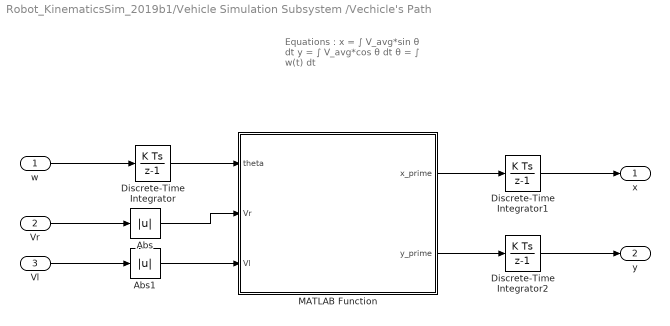
== system Robot_KinematicsSim_2019b1/Vehicle Simulation Subsystem /Vechicle's Path  ==
  note: Equations :
      |
      | x = ∫ V_avg*sin θ dt
      |
      | y = ∫ V_avg*cos θ dt
      |
      | θ = ∫ w(t) dt
  w : Inport
  Vr : Inport  Port=2
  Vl : Inport  Port=3
  Abs : Abs
  Abs1 : Abs
  "Discrete-Time Integrator " : DiscreteIntegrator  SampleTime=-1  ICPrevOutput=DiscIntNeverNeededParam  ICPrevScaledInput=DiscIntNeverNeededParam
  "Discrete-Time Integrator1 " : DiscreteIntegrator  SampleTime=-1  ICPrevOutput=DiscIntNeverNeededParam  ICPrevScaledInput=DiscIntNeverNeededParam
  "Discrete-Time Integrator2 " : DiscreteIntegrator  SampleTime=-1  ICPrevOutput=DiscIntNeverNeededParam  ICPrevScaledInput=DiscIntNeverNeededParam
  "MATLAB Function " : MATLAB Function  TreatAsAtomicUnit=on
  x : Outport
  y : Outport  Port=2
  wires:
  "Discrete-Time Integrator1 "/1 -> x/1
  "Discrete-Time Integrator2 "/1 -> y/1
  "MATLAB Function "/1(x_prime) -> "Discrete-Time Integrator1 "/1
  "MATLAB Function "/2(y_prime) -> "Discrete-Time Integrator2 "/1
  w/1 -> "Discrete-Time Integrator "/1
  "Discrete-Time Integrator "/1 -> "MATLAB Function "/1(theta)
  Vr/1 -> Abs/1
  Abs/1 -> "MATLAB Function "/2(Vr)
  Vl/1 -> Abs1/1
  Abs1/1 -> "MATLAB Function "/3(Vl)

== system Robot_KinematicsSim_2019b1/Vehicle Simulation Subsystem /Vehicle Kinematics model  ==
  note: Equation :
      | w=(Vr-Vl)/L
  Vr : Inport
  L : Inport  Port=2
  "Vl " : Inport  Port=3
  "Add " : Sum  Inputs=+-
  "Convertion to degress per s " : Gain  Gain=180/pi
  "Divide " : Product  Inputs=*/
  "w (in dps) " : Outport
  wires:
  "Vl "/1 -> "Add "/2
  L/1 -> "Divide "/2
  "Divide "/1 -> "Convertion to degress per s "/1
  "Convertion to degress per s "/1 -> "w (in dps) "/1
  Vr/1 -> "Add "/1
  "Add "/1 -> "Divide "/1

== system Robot_KinematicsSim_2019b1/Vehicle Simulation Subsystem 1/Simulation Sensor Subsystem ==
  RWCommand : Inport
  LWCommand : Inport  Port=2
  Conversion to Radians per s : Gain  Gain=2*pi/60
  Conversion to Radians per s1 : Gain  Gain=2*pi/60
  "Wheel Radius in cm " : Gain  Gain=3
  "Wheel Radius in cm1 " : Gain  Gain=3
  Vr : Outport
  Vl : Outport  Port=2
  wires:
  LWCommand/1 -> Conversion to Radians per s1/1
  RWCommand/1 -> Conversion to Radians per s/1
  "Wheel Radius in cm "/1 -> Vr/1
  "Wheel Radius in cm1 "/1 -> Vl/1
  Conversion to Radians per s1/1 -> "Wheel Radius in cm1 "/1
  Conversion to Radians per s/1 -> "Wheel Radius in cm "/1

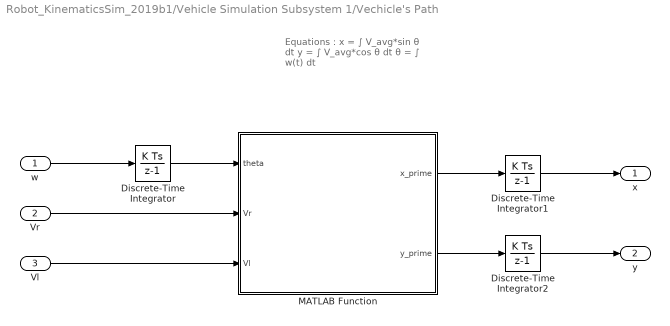
== system Robot_KinematicsSim_2019b1/Vehicle Simulation Subsystem 1/Vechicle's Path  ==
  note: Equations :
      |
      | x = ∫ V_avg*sin θ dt
      |
      | y = ∫ V_avg*cos θ dt
      |
      | θ = ∫ w(t) dt
  w : Inport
  Vr : Inport  Port=2
  Vl : Inport  Port=3
  "Discrete-Time Integrator " : DiscreteIntegrator  SampleTime=-1  ICPrevOutput=DiscIntNeverNeededParam  ICPrevScaledInput=DiscIntNeverNeededParam
  "Discrete-Time Integrator1 " : DiscreteIntegrator  SampleTime=-1  ICPrevOutput=DiscIntNeverNeededParam  ICPrevScaledInput=DiscIntNeverNeededParam
  "Discrete-Time Integrator2 " : DiscreteIntegrator  SampleTime=-1  ICPrevOutput=DiscIntNeverNeededParam  ICPrevScaledInput=DiscIntNeverNeededParam
  "MATLAB Function " : MATLAB Function  TreatAsAtomicUnit=on
  x : Outport
  y : Outport  Port=2
  wires:
  "Discrete-Time Integrator1 "/1 -> x/1
  "Discrete-Time Integrator2 "/1 -> y/1
  "MATLAB Function "/1(x_prime) -> "Discrete-Time Integrator1 "/1
  "MATLAB Function "/2(y_prime) -> "Discrete-Time Integrator2 "/1
  Vl/1 -> "MATLAB Function "/3(Vl)
  Vr/1 -> "MATLAB Function "/2(Vr)
  "Discrete-Time Integrator "/1 -> "MATLAB Function "/1(theta)
  w/1 -> "Discrete-Time Integrator "/1

== system Robot_KinematicsSim_2019b1/Vehicle Simulation Subsystem 1/Vehicle Kinematics model  ==
  note: Equation :
      | w=(Vr-Vl)/L
  Vr : Inport
  L : Inport  Port=2
  "Vl " : Inport  Port=3
  "Add " : Sum  Inputs=+-
  "Convertion to degress per s " : Gain  Gain=180/pi
  "Divide " : Product  Inputs=*/
  "w (in dps) " : Outport
  wires:
  "Vl "/1 -> "Add "/2
  L/1 -> "Divide "/2
  "Divide "/1 -> "Convertion to degress per s "/1
  "Convertion to degress per s "/1 -> "w (in dps) "/1
  Vr/1 -> "Add "/1
  "Add "/1 -> "Divide "/1

== system Robot_KinematicsSim_2019b1/Vehicle Simulation Subsystem2/Simulation Sensor Subsystem ==
  RWCommand : Inport
  LWCommand : Inport  Port=2
  Conversion to Radians per s : Gain  Gain=2*pi/60
  Conversion to Radians per s1 : Gain  Gain=2*pi/60
  "Wheel Radius in cm " : Gain  Gain=3
  "Wheel Radius in cm1 " : Gain  Gain=3
  Vr : Outport
  Vl : Outport  Port=2
  wires:
  Conversion to Radians per s/1 -> "Wheel Radius in cm "/1
  Conversion to Radians per s1/1 -> "Wheel Radius in cm1 "/1
  "Wheel Radius in cm1 "/1 -> Vl/1
  "Wheel Radius in cm "/1 -> Vr/1
  RWCommand/1 -> Conversion to Radians per s/1
  LWCommand/1 -> Conversion to Radians per s1/1

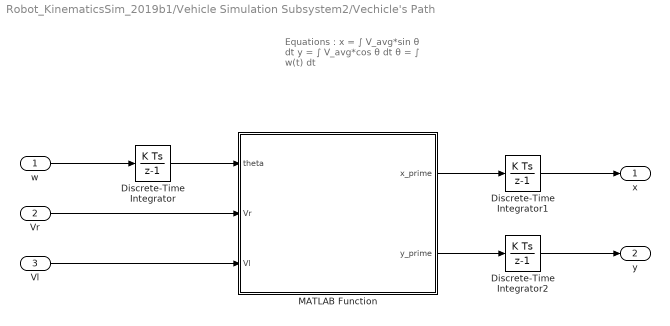
== system Robot_KinematicsSim_2019b1/Vehicle Simulation Subsystem2/Vechicle's Path  ==
  note: Equations :
      |
      | x = ∫ V_avg*sin θ dt
      |
      | y = ∫ V_avg*cos θ dt
      |
      | θ = ∫ w(t) dt
  w : Inport
  Vr : Inport  Port=2
  Vl : Inport  Port=3
  "Discrete-Time Integrator " : DiscreteIntegrator  SampleTime=-1  ICPrevOutput=DiscIntNeverNeededParam  ICPrevScaledInput=DiscIntNeverNeededParam
  "Discrete-Time Integrator1 " : DiscreteIntegrator  SampleTime=-1  ICPrevOutput=DiscIntNeverNeededParam  ICPrevScaledInput=DiscIntNeverNeededParam
  "Discrete-Time Integrator2 " : DiscreteIntegrator  SampleTime=-1  ICPrevOutput=DiscIntNeverNeededParam  ICPrevScaledInput=DiscIntNeverNeededParam
  "MATLAB Function " : MATLAB Function  TreatAsAtomicUnit=on
  x : Outport
  y : Outport  Port=2
  wires:
  w/1 -> "Discrete-Time Integrator "/1
  "Discrete-Time Integrator "/1 -> "MATLAB Function "/1(theta)
  Vr/1 -> "MATLAB Function "/2(Vr)
  Vl/1 -> "MATLAB Function "/3(Vl)
  "MATLAB Function "/2(y_prime) -> "Discrete-Time Integrator2 "/1
  "MATLAB Function "/1(x_prime) -> "Discrete-Time Integrator1 "/1
  "Discrete-Time Integrator2 "/1 -> y/1
  "Discrete-Time Integrator1 "/1 -> x/1

== system Robot_KinematicsSim_2019b1/Vehicle Simulation Subsystem2/Vehicle Kinematics model  ==
  note: Equation :
      | w=(Vr-Vl)/L
  Vr : Inport
  L : Inport  Port=2
  "Vl " : Inport  Port=3
  "Add " : Sum  Inputs=+-
  "Convertion to degress per s " : Gain  Gain=180/pi
  "Divide " : Product  Inputs=*/
  "w (in dps) " : Outport
  wires:
  "Add "/1 -> "Divide "/1
  Vr/1 -> "Add "/1
  "Convertion to degress per s "/1 -> "w (in dps) "/1
  "Divide "/1 -> "Convertion to degress per s "/1
  L/1 -> "Divide "/2
  "Vl "/1 -> "Add "/2

== matlab function Robot_KinematicsSim_2019b1/Path Navigation2/LW Encoder ticks counter ==
  data: encoder_ticks input; encoder_ticks_ud input; y output; count input; reset input
function y = fcn(encoder_ticks,encoder_ticks_ud,count,reset)
    
    if (reset==1)
        count=0;
    end
    if (encoder_ticks~=encoder_ticks_ud)
        count=count+1;
    end
y = count;

== matlab function Robot_KinematicsSim_2019b1/Path Navigation2/RW Encoder ticks counter ==
  data: encoder_ticks input; encoder_ticks_ud input; y output; count input; reset input
function y = fcn(encoder_ticks,encoder_ticks_ud,count,reset)
    
    if (reset==1)
        count=0;
    end
    if (encoder_ticks~=encoder_ticks_ud)
        count=count+1;
    end
y = count;

== matlab function Robot_KinematicsSim_2019b1/Path Navigation2/Speed Control Logic ==
  settings: updateMethod=DISCRETE
  data: LeftEnc input; LeftMtr output; RightEnc input; RightMtr output; out1 output; out2 output; out3 output; out4 output; PIDVal input; TicksLine input; TicksTurn input; res output; Rw input
function [LeftMtr,RightMtr,out1,out2,out3,out4,res] = controlSpeed(LeftEnc,RightEnc,PIDVal,TicksLine,TicksTurn,Rw)
%#codegen
persistent RobotMotion %Variable to keep track of robot state (i.e move straight or take turn)

if isempty(RobotMotion)
    RobotMotion=1; %Initializing variable to the first robot state 1 (i.e first straight motion).Odd values for straight motion and even values for turn
end
res=0;
out1=0;
out2=0;
out3=0;
out4=0;
switch RobotMotion
    case {1} %Checking if the robot state is to take turn
        
        %Check if the encoder count is less than required ticks for turn. Since a delay of 1 sample time is required to 
        %reset the encoder value (due to Unit Delay block in the model), the encoder count value exceeds the required 
        %ticks for straight line for one sample time after the robot state changes for taking turn
        
        if(abs(RightEnc)<(TicksTurn) && abs(LeftEnc)<(TicksTurn))
            LeftMtr=6;
            
            %Same speed is applied to both motors to take turn since the motors are connected in 
            %opposite direction to the robot platform
            RightMtr=6;
            out1=1;
            out2=0;
            out3=0;
            out4=1;
         %   Reset=0;
        else
            LeftMtr=0;
            RightMtr=0;
            RobotMotion=RobotMotion+1; %Changing the robot state to move straight
            
            res=1; %Making the Reset signal to encoder high to reset the encoder
        end
        
    case {2} %Checking if the robot state is to move straight
        
        %Check if the encoder count is less than required ticks for straight line 
        if(abs(LeftEnc)<=TicksLine && abs(RightEnc)<=TicksLine) 
            
            LeftMtr=(abs(Rw)-1); 
            RightMtr=abs(Rw)-1;
            out1=1;
            out2=0;
            out3=1;
            out4=0;
            
        else %Encoder count has exceeded the required ticks for straight line
            
            LeftMtr=0; 
            RightMtr=0;
            RobotMotion=RobotMotion+1; %Changing the robot state to take turn
            res=1; %Making the Reset signal to encoder high to reset the encoder
        end    
        
    otherwise %Robot state is at a value greater than 8 (i.e it has completed tracing the square path)
        LeftMtr=0;
        RightMtr=0;
        res=1;
end
end
